simulink model "hw3s"  (R2020a)
settings: Solver=VariableStepAuto  StartTime=0.0  StopTime=10.0  RelTol=1e-3
values from neighbouring files (symbols this model uses):
  G1 = 1/(j*l)    (= 200)    [hw3.m]
  G2 = l*b + r*j    (= 0.075)    [hw3.m]
  G3 = r*b + K*K    (= 0.2501)    [hw3.m]
  K = 0.01    [hw3.m]    (also in hw4rl.m = 4.23)
  Kd = 20    [hw3.m]
  Ki = 200    [hw3.m]
  Kp = 200    [hw3.m]
settings Model: Creator=izacu  LastModifiedBy=izacu

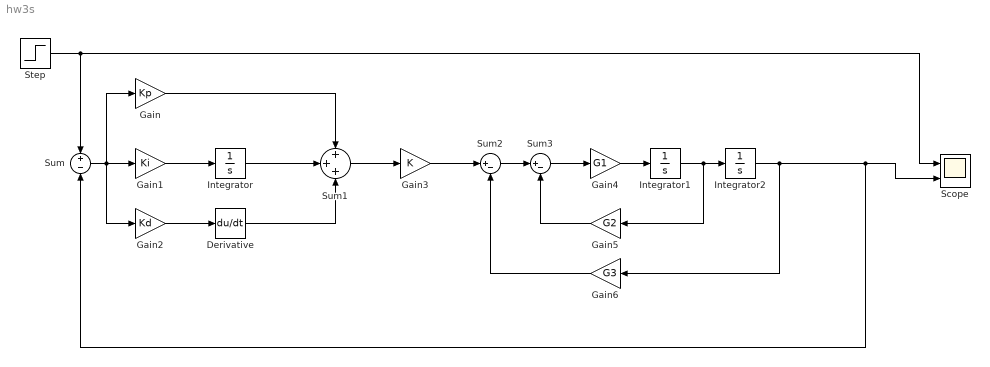
== system hw3s ==
  Derivative : Derivative
  Gain : Gain  Gain=Kp
  Gain1 : Gain  Gain=Ki
  Gain2 : Gain  Gain=Kd
  Gain3 : Gain  Gain=K
  Gain4 : Gain  Gain=G1
  Gain5 : Gain  Gain=G2
  Gain6 : Gain  Gain=G3
  Integrator : Integrator
  Integrator1 : Integrator
  Integrator2 : Integrator
  Scope : Scope  NumInputPorts=2
  Step : Step  After=10  SampleTime=0
  Sum : Sum  Inputs=+-
  Sum1 : Sum  Inputs=+++
  Sum2 : Sum  Inputs=|+-
  Sum3 : Sum  Inputs=|+-
  wires:
  Sum/1 -> Gain2/1, Gain1/1, Gain/1
  Gain1/1 -> Integrator/1
  Integrator/1 -> Sum1/2
  Gain/1 -> Sum1/1
  Gain2/1 -> Derivative/1
  Derivative/1 -> Sum1/3
  Step/1 -> Scope/1, Sum/1
  Sum1/1 -> Gain3/1
  Gain3/1 -> Sum2/1
  Sum2/1 -> Sum3/1
  Sum3/1 -> Gain4/1
  Gain4/1 -> Integrator1/1
  Integrator1/1 -> Integrator2/1, Gain5/1
  Gain5/1 -> Sum3/2
  Integrator2/1 -> Scope/2, Sum/2, Gain6/1
  Gain6/1 -> Sum2/2
